simulink model "optsim"  (Simulink 3.00)
settings: Solver=ode5  SolverMode=SingleTasking  StartTime=0.0  StopTime=100  FixedStep=1  RelTol=1e-3  AbsTol=1e-6
PreLoadFcn:
  | a1=3; a2=43;
PostLoadFcn:
  | optsiminit
values from neighbouring files (symbols this model uses):
  D = sparse(1:n,1:n,d,n,n)    [nlsf1.m]    (also in officeassign.m = triu(D)' + D; optdeblur.m = sparse(mindex,nindex,1/(2*blur+1)))
undefined symbols (not defined in the file or in its folder): I, Kd, Ki, Kp
settings Model: SaveTime=off  TimeSaveName=t  StateSaveName=x  IntegerOverflowMsg=none  Creator=nikita  LastModifiedBy=branch

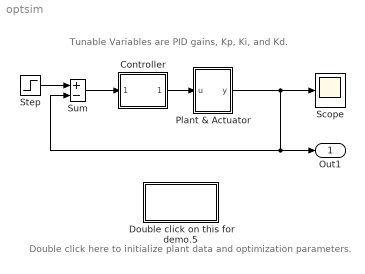
== system optsim ==
  note: Double click here to initialize plant data and optimization parameters.
  note: Tunable Variables are PID gains, Kp, Ki, and Kd.
  Controller : Subsystem  mask(PID Controller){P=Kp,  I=Ki,  D=Kd}
      mask prompts: P "Proportional:";  I "Integral";  D "Derivative:"
      mask help: Enter expressions for proportional, integral, and derivative terms.
      mask Help: This block implements a PID controller where paramaters are entered for the Proportional, Integral and Derivative terms.
      mask Display: disp('PID')
  Double click on this for demo.5 : Subsystem
      settings: OpenFcn=optsiminit
      mask Display: disp('optsiminit')
  Plant & Actuator : Subsystem
  Scope : Scope
      settings: TickLabels=on  TimeRange=100  YMin=0  YMax=1.4  SaveToWorkspace=off  SaveName=ScopeData
  Step : Step  Time=0  Before=0  After=1  SampleTime=0
  Sum : Sum  Inputs=+-  SaturateOnIntegerOverflow=on
  Out1 : Outport  Port=1
  wires:
  Plant & Actuator/1(y) -> Sum/2, Out1/1, Scope/1
  Sum/1 -> Controller/1(In_1)
  Step/1 -> Sum/1
  Controller/1(Out_1) -> Plant & Actuator/1("u ")

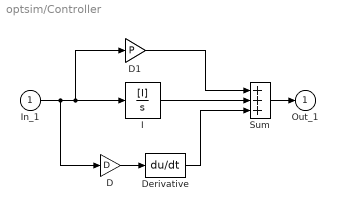
== system optsim/Controller ==
  In_1 : Inport  Port=1  PortWidth=-1  SampleTime=-1  DataType=auto
      settings: SignalType=auto
  D : Gain  Gain=D  SaturateOnIntegerOverflow=on
  D1 : Gain  Gain=P  SaturateOnIntegerOverflow=on
  Derivative : Derivative
  I : TransferFcn  Numerator=[I]  Denominator=[1 0]
  Sum : Sum  Inputs=+++  SaturateOnIntegerOverflow=on
  Out_1 : Outport  Port=1  InitialOutput=0
  wires:
  In_1/1 -> D1/1, I/1, D/1
  Sum/1 -> Out_1/1
  D/1 -> Derivative/1
  Derivative/1 -> Sum/3
  I/1 -> Sum/2
  D1/1 -> Sum/1

== system optsim/Double click on this for demo.5 ==

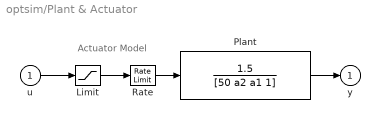
== system optsim/Plant & Actuator ==
  note: Actuator Model
  "u " : Inport  Port=1  PortWidth=-1  SampleTime=-1  DataType=auto
      settings: SignalType=auto
  Limit : Saturate  UpperLimit=2  LowerLimit=-2
  Plant : TransferFcn  Numerator=[1.5]  Denominator=[50 a2 a1 1]
  Rate : RateLimiter  RisingSlewLimit=0.8  FallingSlewLimit=-0.8
  y : Outport  Port=1  InitialOutput=0
  wires:
  Plant/1 -> y/1
  "u "/1 -> Limit/1
  Rate/1 -> Plant/1
  Limit/1 -> Rate/1
